simulink model "SimulinkAnalysisofCheetahTail"  (R2022a)
settings: Solver=ode4  StartTime=0.0  StopTime=1.5  FixedStep=0.001  RelTol=1e-3
undefined symbols (not defined in the file): B_cg_H, B_con_H, B_con_L, bar_len, cd_table, Cf, cl_table, g, gear_ratio, int_point_bar, int_point_tail, ITail, M_add, M_cg_H, M_cg_L, M_cg_W, Mb, Mm, Mt, psi3, rho, T_cg_H, T_fur_gap, T_length, T_width_major, T_width_minor, th2_initial, torque_constant, uncertainty_Forces, uncertainty_Position, Vf, windspeed
(part 14 of 21)

== matlab function SimulinkAnalysisofCheetahTail/Model/Forces/NonConstraintForceMatrix_tail_3 ==
  data: B_con_H parameter; B_con_L parameter; Cd input; Cl input; Q_tail_3 output; M_cg_H parameter; M_cg_L parameter; M_cg_W parameter; T_fur_gap parameter; T_length parameter; T_width_major parameter; T_width_minor parameter; area_tail_3_drag input; bar_len parameter; int_point_tail input; psi3 parameter; rho parameter; windspeed parameter; q input; dq input; ddq input
function Q_tail_3 = NonConstraintForceMatrix_tail_3(B_con_H,B_con_L,Cd,Cl,M_cg_H,M_cg_L,M_cg_W,T_fur_gap,T_length,T_width_major,T_width_minor,area_tail_3_drag,bar_len,int_point_tail,psi3,rho,windspeed,q,dq,ddq)
%#codegen
[x,y,z,phi1,th1,psi1,phi2,th2] = deal(q(1),q(2),q(3),q(4),q(5),q(6),q(7),q(8));
[dx,dy,dz,dphi1,dth1,dpsi1,dphi2,dth2] = deal(dq(1),dq(2),dq(3),dq(4),dq(5),dq(6),dq(7),dq(8));
[ddx,ddy,ddz,ddphi1,ddth1,ddpsi1,ddphi2,ddth2] = deal(ddq(1),ddq(2),ddq(3),ddq(4),ddq(5),ddq(6),ddq(7),ddq(8));
%    This function was generated by the Symbolic Math Toolbox version 9.0.
%    17-Feb-2022 11:27:23

t2 = cos(phi1);
t3 = cos(phi2);
t4 = cos(psi1);
t5 = cos(psi3);
t6 = cos(th1);
t7 = cos(th2);
t8 = sin(phi1);
t9 = sin(phi2);
t10 = sin(psi1);
t11 = sin(psi3);
t12 = sin(th1);
t13 = sin(th2);
t14 = M_cg_L+x;
t15 = M_cg_W+y;
t16 = M_cg_H+z;
t19 = -int_point_tail;
t27 = T_length./2.0;
t28 = bar_len./2.0;
t29 = int_point_tail./2.0;
t17 = B_con_L.*t6;
t18 = B_con_L.*t12;
t20 = t2.*t4;
t21 = t6.*t7;
t22 = t2.*t10;
t23 = t4.*t8;
t24 = t7.*t12;
t25 = t8.*t10;
t26 = t12.*t13;
t30 = B_con_H.*t2.*t6;
t32 = t6.*t14;
t33 = B_con_H.*t2.*t12;
t34 = B_con_H.*t6.*t8;
t37 = t12.*t14;
t39 = -t29;
t42 = t6.*t9.*t13;
t44 = t6.*t10.*t13;
t46 = t8.*t9.*t12;
t49 = t2.*t3.*t6;
t50 = T_length+bar_len+t19;
t53 = t2.*t6.*t9;
t54 = t3.*t6.*t8;
t56 = t2.*t6.*t13;
t57 = t3.*t6.*t13;
t59 = t4.*t6.*t13;
t62 = t3.*t8.*t12;
t63 = t6.*t8.*t9;
t68 = t2.*t6.*t15;
t70 = t2.*t6.*t16;
t73 = t6.*t8.*t15;
t74 = t2.*t12.*t16;
t75 = t6.*t8.*t16;
t77 = t8.*t12.*t15;
t105 = t5.*t6.*t8.*t13;
t111 = t6.*t8.*t11.*t13;
t31 = t4.*t17;
t35 = t4.*t18;
t36 = t10.*t17;
t38 = t10.*t18;
t40 = t2.*t26;
t41 = t3.*t26;
t43 = t9.*t24;
t45 = t10.*t24;
t47 = t12.*t25;
t48 = t9.*t26;
t51 = t2.*t21;
t52 = t4.*t21;
t55 = t12.*t20;
t58 = t3.*t24;
t60 = t4.*t24;
t61 = t10.*t21;
t64 = t12.*t22;
t65 = t12.*t23;
t66 = B_con_H.*t6.*t20;
t67 = t4.*t32;
t69 = B_con_H.*t6.*t22;
t71 = t4.*t37;
t72 = t10.*t32;
t76 = t10.*t37;
t78 = -t33;
t79 = -t34;
t81 = -t46;
t86 = t3.*t6.*t23;
t87 = t13.*t49;
t90 = t3.*t8.*t21;
t91 = t6.*t13.*t20;
t92 = t4.*t57;
t95 = t3.*t6.*t25;
t96 = t6.*t9.*t23;
t97 = t2.*t42;
t99 = t8.*t9.*t21;
t100 = t6.*t13.*t22;
t102 = t3.*t44;
t103 = t4.*t42;
t106 = t6.*t9.*t25;
t110 = t10.*t42;
t113 = -t59;
t116 = t6.*t16.*t20;
t117 = t6.*t15.*t23;
t118 = t6.*t16.*t22;
t119 = t6.*t15.*t25;
t120 = -t68;
t121 = -t73;
t122 = -t74;
t123 = -t75;
t124 = t3.*t20.*t21;
t125 = t3.*t21.*t22;
t126 = t9.*t20.*t21;
t127 = t9.*t21.*t22;
t133 = -t105;
t138 = t24+t56;
t165 = t27+t28+t39;
t80 = -t40;
t82 = -t47;
t83 = -t48;
t84 = t3.*t51;
t85 = t3.*t52;
t88 = t2.*t58;
t89 = t9.*t51;
t93 = t3.*t61;
t94 = t9.*t52;
t98 = t2.*t43;
t101 = t4.*t41;
t104 = t9.*t61;
t107 = -t51;
t108 = t10.*t41;
t109 = t4.*t48;
t112 = -t55;
t114 = -t61;
t115 = t10.*t48;
t129 = -t92;
t131 = -t99;
t136 = -t117;
t137 = -t119;
t139 = t22+t65;
t140 = t23+t64;
t141 = -t124;
t142 = -t125;
t149 = t5.*t138;
t153 = t11.*t138;
t157 = t53+t90;
t161 = t58+t87;
t162 = t60+t91;
t163 = t43+t97;
t164 = t45+t100;
t128 = -t84;
t130 = -t93;
t132 = -t104;
t134 = t4.*t83;
t135 = t10.*t83;
t143 = B_con_H.*t139;
t144 = B_con_H.*t140;
t145 = t21+t80;
t146 = t26+t107;
t147 = t20+t82;
t148 = t25+t112;
t150 = t3.*t139;
t151 = t3.*t140;
t152 = t7.*t140;
t154 = t9.*t139;
t155 = t9.*t140;
t156 = t13.*t140;
t166 = t15.*t139;
t167 = t15.*t140;
t168 = t16.*t139;
t169 = t16.*t140;
t175 = t5.*t13.*t139;
t177 = t11.*t13.*t139;
t185 = -t153;
t189 = t49+t131;
t190 = T_fur_gap.*t157;
t191 = T_fur_gap.*t161;
t192 = int_point_tail.*t157;
t193 = int_point_tail.*t161;
t200 = t5.*t162;
t201 = t11.*t162;
t202 = t5.*t163;
t203 = t5.*t164;
t204 = t11.*t163;
t205 = t11.*t164;
t228 = t42+t62+t98;
t231 = t57+t81+t88;
t232 = t54+t83+t89;
t266 = t96+t101+t141;
t268 = t106+t108+t142;
t282 = t157.*t165;
t283 = t161.*t165;
t158 = B_con_H.*t147;
t159 = B_con_H.*t148;
t160 = -t144;
t170 = t7.*t150;
t171 = t7.*t151;
t172 = t13.*t151;
t173 = t7.*t154;
t174 = t9.*t152;
t176 = t13.*t155;
t178 = t5.*t145;
t179 = t5.*t146;
t180 = t3.*t147;
t181 = t3.*t148;
t182 = t7.*t148;
t183 = t11.*t145;
t184 = t11.*t146;
t186 = t9.*t147;
t187 = t9.*t148;
t188 = t13.*t148;
t194 = t15.*t147;
t195 = t15.*t148;
t196 = -t167;
t197 = t16.*t147;
t198 = t16.*t148;
t199 = -t169;
t212 = t5.*t13.*t147;
t214 = t11.*t13.*t147;
t215 = -t177;
t221 = t5.*t189;
t222 = t11.*t189;
t223 = -t205;
t227 = t44+t152;
t229 = t114+t156;
t230 = t41+t63+t128;
t236 = t5.*t228;
t237 = t11.*t228;
t239 = T_fur_gap.*t231;
t240 = T_fur_gap.*t232;
t242 = int_point_tail.*t231;
t243 = int_point_tail.*t232;
t246 = -t5.*(t61-t156);
t249 = -t11.*(t61-t156);
t250 = t5.*t232;
t252 = t11.*t232;
t267 = t86+t126+t134;
t269 = t95+t127+t135;
t276 = T_fur_gap.*t266;
t277 = int_point_tail.*t266;
t278 = T_fur_gap.*t268;
t279 = int_point_tail.*t268;
t303 = t165.*t231;
t304 = t165.*t232;
t325 = t165.*t266;
t326 = t165.*t268;
t370 = t191+t193+t283;
t397 = t79+t120+t123+t190+t192+t282;
t206 = t7.*t180;
t207 = t7.*t181;
t208 = -t170;
t209 = t13.*t181;
t210 = t7.*t186;
t211 = t9.*t182;
t213 = t13.*t187;
t216 = -t178;
t217 = -t180;
t218 = -t184;
t219 = -t194;
t220 = -t195;
t226 = -t214;
t233 = t52+t188;
t234 = t5.*t227;
t235 = t11.*t227;
t238 = T_fur_gap.*t230;
t241 = int_point_tail.*t230;
t244 = t113+t182;
t251 = t12.*t230;
t254 = t130+t172;
t256 = t132+t176;
t257 = t2.*t6.*t230;
t258 = -t5.*(t59-t182);
t259 = t6.*t8.*t230;
t260 = -t11.*(t59-t182);
t262 = -T_fur_gap.*(t93-t172);
t264 = -int_point_tail.*(t93-t172);
t265 = t111+t221;
t270 = -t5.*(t104-t176);
t272 = -t11.*(t104-t176);
t274 = t5.*(t59-t182);
t280 = t133+t222;
t281 = t5.*t269;
t284 = t11.*t269;
t285 = t5.*t267;
t286 = t11.*t267;
t288 = t173+t181;
t290 = t179+t204;
t298 = -T_fur_gap.*(t170-t187);
t300 = -int_point_tail.*(t170-t187);
t302 = t165.*t230;
t305 = t149+t252;
t306 = t102+t171+t186;
t307 = t183+t236;
t311 = t185+t250;
t316 = -t165.*(t93-t172);
t333 = -t12.*(t153-t250);
t339 = -t2.*t6.*(t153-t250);
t340 = -t6.*t8.*(t153-t250);
t346 = t2.*t6.*(t153-t250);
t350 = -t165.*(t170-t187);
t395 = t240+t243+t304;
t396 = t230.*t370;
t401 = -t370.*(t153-t250);
t402 = t370.*(t153-t250);
t404 = -t230.*(t34+t68+t75-t190-t192-t282);
t408 = t17+t32+t77+t78+t122+t239+t242+t303;
t416 = (t153-t250).*(t34+t68+t75-t190-t192-t282);
t432 = t38+t69+t76+t118+t137+t278+t279+t326;
t433 = t35+t66+t71+t116+t136+t276+t277+t325;
t224 = -t206;
t225 = -t211;
t245 = t5.*t233;
t247 = t11.*t233;
t248 = -t234;
t253 = t85+t209;
t255 = t94+t213;
t273 = -t257;
t287 = t151+t210;
t289 = -t285;
t292 = t187+t208;
t294 = t5.*t288;
t296 = t11.*t288;
t301 = t202+t218;
t308 = T_fur_gap.*t306;
t309 = int_point_tail.*t306;
t310 = t129+t154+t207;
t313 = t216+t237;
t314 = t110+t174+t217;
t317 = t12.*t305;
t319 = t5.*t306.*windspeed;
t327 = t2.*t6.*t305;
t328 = t6.*t8.*t305;
t329 = t6.*t10.*t306;
t347 = t200+t286;
t348 = t203+t284;
t352 = t223+t281;
t354 = t140.*t306;
t355 = t235+t270;
t359 = t147.*t306;
t363 = t165.*t306;
t399 = t262+t264+t316;
t400 = t305.*t370;
t403 = t230.*t395;
t406 = t18+t30+t37+t70+t121+t238+t241+t302;
t413 = t305.*t395;
t414 = -t305.*(t34+t68+t75-t190-t192-t282);
t415 = -t395.*(t153-t250);
t417 = t395.*(t153-t250);
t420 = -t416;
t427 = -t306.*(T_fur_gap.*(t93-t172)+int_point_tail.*(t93-t172)+t165.*(t93-t172));
t431 = t306.*(T_fur_gap.*(t93-t172)+int_point_tail.*(t93-t172)+t165.*(t93-t172));
t439 = t230.*t408;
t452 = t305.*t408;
t453 = -t408.*(t153-t250);
t455 = t408.*(t153-t250);
t456 = t143+t168+t220+t298+t300+t350;
t462 = t306.*t432;
t261 = T_fur_gap.*t253;
t263 = int_point_tail.*t253;
t271 = t11.*t255;
t275 = t5.*t255;
t291 = t155+t224;
t293 = t5.*t287;
t295 = t11.*t287;
t312 = t103+t150+t225;
t315 = t165.*t253;
t318 = T_fur_gap.*t310;
t321 = int_point_tail.*t310;
t322 = T_fur_gap.*t314;
t324 = int_point_tail.*t314;
t331 = t5.*t314;
t334 = t11.*t314;
t336 = t11.*t310.*windspeed;
t337 = t19.*t310;
t338 = t4.*t6.*t310;
t341 = -t328;
t351 = t201+t289;
t353 = t175+t296;
t356 = t215+t294;
t358 = t139.*t310;
t360 = t248+t272;
t362 = t148.*t310;
t365 = t165.*t310;
t367 = t165.*t314;
t405 = -t403;
t418 = t157.*t406;
t419 = t161.*t406;
t428 = t231.*t406;
t429 = t232.*t406;
t434 = t5.*t230.*t406;
t435 = t11.*t230.*t406;
t441 = -t439;
t444 = t265.*t406;
t445 = -t406.*(t105-t222);
t447 = t290.*t406;
t448 = -t406.*(t184-t202);
t450 = t307.*t406;
t451 = -t406.*(t178-t237);
t454 = -t452;
t463 = t310.*t433;
t476 = t36+t72+t160+t199+t219+t308+t309+t363;
t478 = -t310.*(-t143-t168+t195+T_fur_gap.*(t170-t187)+int_point_tail.*(t170-t187)+t165.*(t170-t187));
t480 = t310.*(-t143-t168+t195+T_fur_gap.*(t170-t187)+int_point_tail.*(t170-t187)+t165.*(t170-t187));
t297 = T_fur_gap.*t291;
t299 = int_point_tail.*t291;
t320 = T_fur_gap.*t312;
t323 = int_point_tail.*t312;
t330 = t5.*t312;
t332 = t11.*t312;
t335 = -t318;
t342 = -t331;
t344 = -t336;
t345 = -t338;
t349 = t165.*t291;
t357 = t212+t295;
t361 = t226+t293;
t364 = t260+t275;
t366 = t165.*t312;
t368 = t271+t274;
t369 = -t365;
t372 = t246+t334;
t375 = t5.*windspeed.*(t334-t5.*(t61-t156));
t378 = t6.*t10.*(t334-t5.*(t61-t156));
t379 = -t5.*windspeed.*(t331+t11.*(t61-t156));
t384 = -t6.*t10.*(t331+t11.*(t61-t156));
t388 = t140.*(t334-t5.*(t61-t156));
t391 = t147.*(t334-t5.*(t61-t156));
t392 = -t140.*(t331+t11.*(t61-t156));
t394 = -t147.*(t331+t11.*(t61-t156));
t398 = t261+t263+t315;
t421 = t259+t358+t359;
t424 = t273+t354+t362;
t436 = -t428;
t437 = -t429;
t440 = -t435;
t443 = t322+t324+t367;
t446 = -t444;
t449 = -t447;
t459 = -(t334-t5.*(t61-t156)).*(T_fur_gap.*(t93-t172)+int_point_tail.*(t93-t172)+t165.*(t93-t172));
t461 = (t331+t11.*(t61-t156)).*(T_fur_gap.*(t93-t172)+int_point_tail.*(t93-t172)+t165.*(t93-t172));
t465 = -t463;
t482 = t432.*(t334-t5.*(t61-t156));
t485 = -t432.*(t331+t11.*(t61-t156));
t506 = -t476.*(t93-t172);
t507 = t476.*(t93-t172);
t508 = t268.*t476;
t510 = t291.*t476;
t518 = t5.*t306.*t476;
t519 = t11.*t306.*t476;
t520 = t314.*t476;
t522 = t348.*t476;
t524 = -t476.*(t205-t281);
t528 = t355.*t476;
t530 = -t476.*(t234+t11.*(t104-t176));
t532 = -t476.*(t214-t293);
t343 = -t332;
t371 = t247+t330;
t374 = t249+t342;
t385 = -t378;
t407 = t251+t329+t345;
t422 = ddy.*t421;
t423 = dy.*t421;
t425 = ddz.*t424;
t426 = dz.*t424;
t430 = t310.*t398;
t442 = t320+t323+t366;
t458 = t158+t196+t197+t297+t299+t349;
t464 = t306.*t443;
t477 = t31+t67+t159+t166+t198+t335+t337+t369;
t486 = -t482;
t493 = t443.*(t334-t5.*(t61-t156));
t500 = -t443.*(t331+t11.*(t61-t156));
t512 = -t510;
t521 = -t519;
t529 = t357.*t476;
t531 = -t528;
t373 = t245+t343;
t376 = t11.*t371.*windspeed;
t377 = t4.*t6.*t371;
t387 = t139.*t371;
t389 = t148.*t371;
t409 = ddx.*t407;
t410 = dx.*t407;
t438 = -t430;
t457 = t371.*t398;
t466 = t310.*t442;
t479 = t306.*t458;
t483 = t371.*t433;
t494 = t371.*t442;
t509 = t253.*t477;
t511 = t266.*t477;
t513 = -t371.*(-t143-t168+t195+T_fur_gap.*(t170-t187)+int_point_tail.*(t170-t187)+t165.*(t170-t187));
t515 = t458.*(t334-t5.*(t61-t156));
t516 = -t458.*(t331+t11.*(t61-t156));
t517 = -t477.*(t170-t187);
t523 = t312.*t477;
t525 = t5.*t310.*t477;
t526 = t11.*t310.*t477;
t533 = -t529;
t534 = t347.*t477;
t535 = t351.*t477;
t536 = t353.*t477;
t538 = -t477.*(t177-t294);
t539 = t477.*(t177-t294);
t540 = t364.*t477;
t541 = t368.*t477;
Q_tail_3 = ft_1({Cd,Cl,T_fur_gap,T_width_major,T_width_minor,area_tail_3_drag,ddphi1,ddphi2,ddth1,ddth2,ddx,ddy,ddz,dphi1,dphi2,dth1,dth2,dx,dy,dz,int_point_tail,rho,t10,t104,t105,t11,t12,t138,t139,t140,t143,t147,t148,t153,t156,t165,t168,t170,t172,t176,t178,t187,t190,t192,t195,t2,t205,t214,t222,t230,t232,t233,t234,t237,t250,t281,t282,t293,t305,t306,t310,t312,t314,t317,t319,t327,t331,t333,t334,t34,t340,t341,t344,t346,t370,t371,t373,t375,t376,t377,t379,t384,t385,t387,t388,t389,t391,t392,t394,t395,t396,t398,t4,t400,t402,t403,t404,t405,t406,t408,t409,t410,t413,t414,t415,t416,t417,t418,t419,t420,t422,t423,t425,t426,t428,t429,t431,t432,t433,t434,t436,t437,t438,t439,t440,t441,t442,t443,t444,t445,t446,t447,t448,t449,t450,t451,t452,t453,t454,t455,t457,t458,t459,t461,t462,t463,t464,t465,t466,t476,t477,t478,t479,t480,t482,t483,t485,t486,t493,t494,t5,t50,t500,t507,t508,t509,t510,t511,t512,t513,t515,t516,t517,t518,t520,t521,t522,t523,t524,t525,t526,t529,t530,t531,t532,t533,t534,t535,t536,t538,t539,t540,t541,t6,t61,t68,t75,t8,t93,th2,windspeed});
end
function Q_tail_3 = ft_1(ct)
Cd = ct{1};
Cl = ct{2};
T_fur_gap = ct{3};
T_width_major = ct{4};
T_width_minor = ct{5};
area_tail_3_drag = ct{6};
ddphi1 = ct{7};
ddphi2 = ct{8};
ddth1 = ct{9};
ddth2 = ct{10};
ddx = ct{11};
ddy = ct{12};
ddz = ct{13};
dphi1 = ct{14};
dphi2 = ct{15};
dth1 = ct{16};
dth2 = ct{17};
dx = ct{18};
dy = ct{19};
dz = ct{20};
int_point_tail = ct{21};
rho = ct{22};
t10 = ct{23};
t104 = ct{24};
t105 = ct{25};
t11 = ct{26};
t12 = ct{27};
t138 = ct{28};
t139 = ct{29};
t140 = ct{30};
t143 = ct{31};
t147 = ct{32};
t148 = ct{33};
t153 = ct{34};
t156 = ct{35};
t165 = ct{36};
t168 = ct{37};
t170 = ct{38};
t172 = ct{39};
t176 = ct{40};
t178 = ct{41};
t187 = ct{42};
t190 = ct{43};
t192 = ct{44};
t195 = ct{45};
t2 = ct{46};
t205 = ct{47};
t214 = ct{48};
t222 = ct{49};
t230 = ct{50};
t232 = ct{51};
t233 = ct{52};
t234 = ct{53};
t237 = ct{54};
t250 = ct{55};
t281 = ct{56};
t282 = ct{57};
t293 = ct{58};
t305 = ct{59};
t306 = ct{60};
t310 = ct{61};
t312 = ct{62};
t314 = ct{63};
t317 = ct{64};
t319 = ct{65};
t327 = ct{66};
t331 = ct{67};
t333 = ct{68};
t334 = ct{69};
t34 = ct{70};
t340 = ct{71};
t341 = ct{72};
t344 = ct{73};
t346 = ct{74};
t370 = ct{75};
t371 = ct{76};
t373 = ct{77};
t375 = ct{78};
t376 = ct{79};
t377 = ct{80};
t379 = ct{81};
t384 = ct{82};
t385 = ct{83};
t387 = ct{84};
t388 = ct{85};
t389 = ct{86};
t391 = ct{87};
t392 = ct{88};
t394 = ct{89};
t395 = ct{90};
t396 = ct{91};
t398 = ct{92};
t4 = ct{93};
t400 = ct{94};
t402 = ct{95};
t403 = ct{96};
t404 = ct{97};
t405 = ct{98};
t406 = ct{99};
t408 = ct{100};
t409 = ct{101};
t410 = ct{102};
t413 = ct{103};
t414 = ct{104};
t415 = ct{105};
t416 = ct{106};
t417 = ct{107};
t418 = ct{108};
t419 = ct{109};
t420 = ct{110};
t422 = ct{111};
t423 = ct{112};
t425 = ct{113};
t426 = ct{114};
t428 = ct{115};
t429 = ct{116};
t431 = ct{117};
t432 = ct{118};
t433 = ct{119};
t434 = ct{120};
t436 = ct{121};
t437 = ct{122};
t438 = ct{123};
t439 = ct{124};
t440 = ct{125};
t441 = ct{126};
t442 = ct{127};
t443 = ct{128};
t444 = ct{129};
t445 = ct{130};
t446 = ct{131};
t447 = ct{132};
t448 = ct{133};
t449 = ct{134};
t450 = ct{135};
t451 = ct{136};
t452 = ct{137};
t453 = ct{138};
t454 = ct{139};
t455 = ct{140};
t457 = ct{141};
t458 = ct{142};
t459 = ct{143};
t461 = ct{144};
t462 = ct{145};
t463 = ct{146};
t464 = ct{147};
t465 = ct{148};
t466 = ct{149};
t476 = ct{150};
t477 = ct{151};
t478 = ct{152};
t479 = ct{153};
t480 = ct{154};
t482 = ct{155};
t483 = ct{156};
t485 = ct{157};
t486 = ct{158};
t493 = ct{159};
t494 = ct{160};
t5 = ct{161};
t50 = ct{162};
t500 = ct{163};
t507 = ct{164};
t508 = ct{165};
t509 = ct{166};
t510 = ct{167};
t511 = ct{168};
t512 = ct{169};
t513 = ct{170};
t515 = ct{171};
t516 = ct{172};
t517 = ct{173};
t518 = ct{174};
t520 = ct{175};
t521 = ct{176};
t522 = ct{177};
t523 = ct{178};
t524 = ct{179};
t525 = ct{180};
t526 = ct{181};
t529 = ct{182};
t530 = ct{183};
t531 = ct{184};
t532 = ct{185};
t533 = ct{186};
t534 = ct{187};
t535 = ct{188};
t536 = ct{189};
t538 = ct{190};
t539 = ct{191};
t540 = ct{192};
t541 = ct{193};
t6 = ct{194};
t61 = ct{195};
t68 = ct{196};
t75 = ct{197};
t8 = ct{198};
t93 = ct{199};
th2 = ct{200};
windspeed = ct{201};
t380 = t11.*t373.*windspeed;
t381 = -t376;
t382 = t4.*t6.*t373;
t383 = -t377;
t390 = t139.*t373;
t393 = t148.*t373;
t411 = -t409;
t412 = -t410;
t460 = t373.*t398;
t467 = -t466;
t472 = -ddx.*(t377+t12.*(t153-t250)+t6.*t10.*(t331+t11.*(t61-t156)));
t473 = -dx.*(t377+t12.*(t153-t250)+t6.*t10.*(t331+t11.*(t61-t156)));
t474 = ddx.*(t377+t12.*(t153-t250)+t6.*t10.*(t331+t11.*(t61-t156)));
t475 = dx.*(t377+t12.*(t153-t250)+t6.*t10.*(t331+t11.*(t61-t156)));
t481 = -t479;
t487 = t373.*t433;
t488 = -t483;
t489 = t340+t387+t394;
t495 = -ddy.*(-t387+t147.*(t331+t11.*(t61-t156))+t6.*t8.*(t153-t250));
t497 = -dy.*(-t387+t147.*(t331+t11.*(t61-t156))+t6.*t8.*(t153-t250));
t499 = t346+t389+t392;
t501 = t373.*t442;
t502 = -t494;
t514 = -t373.*(-t143-t168+t195+T_fur_gap.*(t170-t187)+int_point_tail.*(t170-t187)+t165.*(t170-t187));
t527 = -t525;
t537 = -t535;
t542 = -t541;
t543 = t396+t419+t431+t438+t507+t509;
t548 = t436+t441+t462+t465+t508+t511;
t549 = -ddth1.*(t428+t439-t462+t463-t508-t511);
t550 = -dth1.*(t428+t439-t462+t463-t508-t511);
t552 = t402+t448+t457+t461+t531+t540;
t554 = -ddphi2.*(t403+t429-t464+t466-t520-t523);
t555 = -dphi2.*(t403+t429-t464+t466-t520-t523);
t561 = -ddphi1.*(-t418+t478+t479+t510+t230.*(t34+t68+t75-t190-t192-t282)+t477.*(t170-t187));
t562 = -dphi1.*(-t418+t478+t479+t510+t230.*(t34+t68+t75-t190-t192-t282)+t477.*(t170-t187));
t563 = ddphi1.*(-t418+t478+t479+t510+t230.*(t34+t68+t75-t190-t192-t282)+t477.*(t170-t187));
t564 = dphi1.*(-t418+t478+t479+t510+t230.*(t34+t68+t75-t190-t192-t282)+t477.*(t170-t187));
t569 = -ddphi2.*(t415-t434+t494-t518+t525+t443.*(t331+t11.*(t61-t156)));
t570 = -dphi2.*(t415-t434+t494-t518+t525+t443.*(t331+t11.*(t61-t156)));
t577 = -ddth1.*(-t450+t453+t483+t535+t432.*(t331+t11.*(t61-t156))+t476.*(t205-t281));
t578 = -dth1.*(-t450+t453+t483+t535+t432.*(t331+t11.*(t61-t156))+t476.*(t205-t281));
t580 = -ddphi1.*(-t515+t529-t536+t305.*(t34+t68+t75-t190-t192-t282)+t406.*(t105-t222)+t373.*(-t143-t168+t195+T_fur_gap.*(t170-t187)+int_point_tail.*(t170-t187)+t165.*(t170-t187)));
t581 = -dphi1.*(-t515+t529-t536+t305.*(t34+t68+t75-t190-t192-t282)+t406.*(t105-t222)+t373.*(-t143-t168+t195+T_fur_gap.*(t170-t187)+int_point_tail.*(t170-t187)+t165.*(t170-t187)));
t582 = t420+t446+t513+t516+t532+t539;
t583 = -ddphi1.*(t416+t444+t538+t458.*(t331+t11.*(t61-t156))+t476.*(t214-t293)+t371.*(-t143-t168+t195+T_fur_gap.*(t170-t187)+int_point_tail.*(t170-t187)+t165.*(t170-t187)));
t584 = -dphi1.*(t416+t444+t538+t458.*(t331+t11.*(t61-t156))+t476.*(t214-t293)+t371.*(-t143-t168+t195+T_fur_gap.*(t170-t187)+int_point_tail.*(t170-t187)+t165.*(t170-t187)));
t386 = -t380;
t468 = t317+t382+t385;
t471 = t333+t383+t384;
t484 = t327+t388+t393;
t490 = t341+t390+t391;
t503 = ddz.*t499;
t504 = dz.*t499;
t505 = -t501;
t544 = ddth2.*t543;
t545 = dth2.*t543;
t551 = t405+t437+t464+t467+t520+t523;
t553 = t400+t449+t459+t460+t530+t542;
t556 = ddth2.*t552;
t557 = -ddth2.*(-t400+t447-t460+t541+t476.*(t234+t11.*(t104-t176))+(t334-t5.*(t61-t156)).*(T_fur_gap.*(t93-t172)+int_point_tail.*(t93-t172)+t165.*(t93-t172)));
t558 = dth2.*t552;
t559 = -dth2.*(-t400+t447-t460+t541+t476.*(t234+t11.*(t104-t176))+(t334-t5.*(t61-t156)).*(T_fur_gap.*(t93-t172)+int_point_tail.*(t93-t172)+t165.*(t93-t172)));
t560 = t404+t418+t480+t481+t512+t517;
t568 = t417+t434+t500+t502+t518+t527;
t571 = t451+t454+t486+t487+t522+t534;
t572 = -ddth1.*(t452+t482-t487-t522-t534+t406.*(t178-t237));
t573 = -dth1.*(t452+t482-t487-t522-t534+t406.*(t178-t237));
t574 = ddth1.*(t452+t482-t487-t522-t534+t406.*(t178-t237));
t575 = dth1.*(t452+t482-t487-t522-t534+t406.*(t178-t237));
t576 = t450+t455+t485+t488+t524+t537;
t579 = t414+t445+t514+t515+t533+t536;
t469 = ddx.*t468;
t470 = dx.*t468;
t491 = ddz.*t484;
t492 = dz.*t484;
t496 = ddy.*t490;
t498 = dy.*t490;
t546 = -t544;
t547 = -t545;
t565 = t413+t440+t493+t505+t521+t526;
t594 = t474+t495+t503+t556+t569+t577+t583;
t600 = t379+t381+t475+t497+t504+t558+t570+t578+t584;
t602 = -1.0./(t376+t473-t504-t558+dy.*(-t387+t147.*(t331+t11.*(t61-t156))+t6.*t8.*(t153-t250))+dphi2.*(t415-t434+t494-t518+t525+t443.*(t331+t11.*(t61-t156)))+dphi1.*(t416+t444+t538+t458.*(t331+t11.*(t61-t156))+t476.*(t214-t293)+t371.*(-t143-t168+t195+T_fur_gap.*(t170-t187)+int_point_tail.*(t170-t187)+t165.*(t170-t187)))+dth1.*(-t450+t453+t483+t535+t432.*(t331+t11.*(t61-t156))+t476.*(t205-t281))+t5.*windspeed.*(t331+t11.*(t61-t156)));
t566 = ddphi2.*t565;
t567 = dphi2.*t565;
t585 = t411+t422+t425+t546+t549+t554+t563;
t588 = t319+t344+t412+t423+t426+t547+t550+t555+t564;
t595 = abs(t594);
t601 = abs(t600);
t586 = abs(t585);
t589 = abs(t588);
t591 = t469+t491+t496+t557+t566+t574+t580;
t596 = t595.^2;
t597 = t375+t386+t470+t492+t498+t559+t567+t575+t581;
t603 = t601.^2;
t604 = t588.*t602;
t587 = t586.^2;
t590 = t589.^2;
t592 = abs(t591);
t598 = abs(t597);
t605 = atan(t604);
t593 = t592.^2;
t599 = t598.^2;
t606 = -t605;
t607 = t606+th2;
t609 = t587+t593+t596;
t612 = t590+t599+t603;
t608 = cos(t607);
t610 = sqrt(t609);
t613 = sqrt(t612);
t611 = (T_width_major.*T_width_minor.*rho.*t50.*t610.*pi)./2.0e+1;
t614 = 1.0./t613;
t615 = (Cd.*area_tail_3_drag.*rho.*t608.*t612)./2.0;
t616 = (Cl.*T_width_major.*T_width_minor.*rho.*t588.*t608.*t613.*pi)./2.0;
t617 = Cl.*T_width_major.*T_width_minor.*rho.*t588.*t608.*t613.*pi.*3.061616997868383e-17;
t618 = (Cl.*T_width_major.*T_width_minor.*rho.*t138.*t597.*t608.*t613.*pi)./2.0;
t619 = Cl.*T_width_major.*T_width_minor.*rho.*t608.*t613.*pi.*(t376+t473-t504-t558+dy.*(-t387+t147.*(t331+t11.*(t61-t156))+t6.*t8.*(t153-t250))+dphi2.*(t415-t434+t494-t518+t525+t443.*(t331+t11.*(t61-t156)))+dphi1.*(t416+t444+t538+t458.*(t331+t11.*(t61-t156))+t476.*(t214-t293)+t371.*(-t143-t168+t195+T_fur_gap.*(t170-t187)+int_point_tail.*(t170-t187)+t165.*(t170-t187)))+dth1.*(-t450+t453+t483+t535+t432.*(t331+t11.*(t61-t156))+t476.*(t205-t281))+t5.*windspeed.*(t331+t11.*(t61-t156))).*(-1.0./2.0);
t620 = (Cl.*T_width_major.*T_width_minor.*rho.*t233.*t597.*t608.*t613.*pi)./2.0;
t621 = Cl.*T_width_major.*T_width_minor.*rho.*t597.*t608.*t613.*pi.*(t61-t156).*(-1.0./2.0);
et1 = Cl.*T_width_major.*T_width_minor.*rho.*t608.*t613.*pi.*(t376+t473-t504-t558+dy.*(-t387+t147.*(t331+t11.*(t61-t156))+t6.*t8.*(t153-t250))+dphi2.*(t415-t434+t494-t518+t525+t443.*(t331+t11.*(t61-t156)))+dphi1.*(t416+t444+t538+t458.*(t331+t11.*(t61-t156))+t476.*(t214-t293)+t371.*(-t143-t168+t195+T_fur_gap.*(t170-t187)+int_point_tail.*(t170-t187)+t165.*(t170-t187)))+dth1.*(-t450+t453+t483+t535+t432.*(t331+t11.*(t61-t156))+t476.*(t205-t281))+t5.*windspeed.*(t331+t11.*(t61-t156)));
et2 = -3.061616997868383e-17;
t622 = et1.*et2;
et3 = Cl.*T_width_major.*T_width_minor.*rho.*t608.*t613.*pi.*(t376+t473-t504-t558+dy.*(-t387+t147.*(t331+t11.*(t61-t156))+t6.*t8.*(t153-t250))+dphi2.*(t415-t434+t494-t518+t525+t443.*(t331+t11.*(t61-t156)))+dphi1.*(t416+t444+t538+t458.*(t331+t11.*(t61-t156))+t476.*(t214-t293)+t371.*(-t143-t168+t195+T_fur_gap.*(t170-t187)+int_point_tail.*(t170-t187)+t165.*(t170-t187)))+dth1.*(-t450+t453+t483+t535+t432.*(t331+t11.*(t61-t156))+t476.*(t205-t281))+t5.*windspeed.*(t331+t11.*(t61-t156)));
et4 = 3.061616997868383e-17;
t623 = et3.*et4;
t624 = t611+t615;
t628 = t617+t619;
t629 = t616+t623;
t625 = t230.*t588.*t614.*t624;
t626 = t306.*t588.*t614.*t624;
t627 = t310.*t588.*t614.*t624;
t630 = t230.*t628;
t631 = t232.*t629;
t633 = t306.*t628;
t634 = t310.*t628;
t635 = t312.*t629;
t636 = t314.*t629;
t638 = t138.*t597.*t614.*t624;
t640 = t233.*t597.*t614.*t624;
t641 = -t597.*t614.*t624.*(t61-t156);
t642 = -t232.*t614.*t624.*(t376+t473-t504-t558+dy.*(-t387+t147.*(t331+t11.*(t61-t156))+t6.*t8.*(t153-t250))+dphi2.*(t415-t434+t494-t518+t525+t443.*(t331+t11.*(t61-t156)))+dphi1.*(t416+t444+t538+t458.*(t331+t11.*(t61-t156))+t476.*(t214-t293)+t371.*(-t143-t168+t195+T_fur_gap.*(t170-t187)+int_point_tail.*(t170-t187)+t165.*(t170-t187)))+dth1.*(-t450+t453+t483+t535+t432.*(t331+t11.*(t61-t156))+t476.*(t205-t281))+t5.*windspeed.*(t331+t11.*(t61-t156)));
t643 = -t312.*t614.*t624.*(t376+t473-t504-t558+dy.*(-t387+t147.*(t331+t11.*(t61-t156))+t6.*t8.*(t153-t250))+dphi2.*(t415-t434+t494-t518+t525+t443.*(t331+t11.*(t61-t156)))+dphi1.*(t416+t444+t538+t458.*(t331+t11.*(t61-t156))+t476.*(t214-t293)+t371.*(-t143-t168+t195+T_fur_gap.*(t170-t187)+int_point_tail.*(t170-t187)+t165.*(t170-t187)))+dth1.*(-t450+t453+t483+t535+t432.*(t331+t11.*(t61-t156))+t476.*(t205-t281))+t5.*windspeed.*(t331+t11.*(t61-t156)));
t644 = -t314.*t614.*t624.*(t376+t473-t504-t558+dy.*(-t387+t147.*(t331+t11.*(t61-t156))+t6.*t8.*(t153-t250))+dphi2.*(t415-t434+t494-t518+t525+t443.*(t331+t11.*(t61-t156)))+dphi1.*(t416+t444+t538+t458.*(t331+t11.*(t61-t156))+t476.*(t214-t293)+t371.*(-t143-t168+t195+T_fur_gap.*(t170-t187)+int_point_tail.*(t170-t187)+t165.*(t170-t187)))+dth1.*(-t450+t453+t483+t535+t432.*(t331+t11.*(t61-t156))+t476.*(t205-t281))+t5.*windspeed.*(t331+t11.*(t61-t156)));
t645 = t314.*t614.*t624.*(t376+t473-t504-t558+dy.*(-t387+t147.*(t331+t11.*(t61-t156))+t6.*t8.*(t153-t250))+dphi2.*(t415-t434+t494-t518+t525+t443.*(t331+t11.*(t61-t156)))+dphi1.*(t416+t444+t538+t458.*(t331+t11.*(t61-t156))+t476.*(t214-t293)+t371.*(-t143-t168+t195+T_fur_gap.*(t170-t187)+int_point_tail.*(t170-t187)+t165.*(t170-t187)))+dth1.*(-t450+t453+t483+t535+t432.*(t331+t11.*(t61-t156))+t476.*(t205-t281))+t5.*windspeed.*(t331+t11.*(t61-t156)));
t632 = -t630;
t637 = -t635;
t639 = -t638;
t647 = t621+t633+t636;
t650 = t627+t640+t643;
t651 = t626+t641+t645;
t646 = t618+t631+t632;
t648 = t620+t634+t637;
t649 = t625+t639+t642;
et5 = -t12.*t646+t12.*(-t625+t638+t232.*t614.*t624.*(t376+t473-t504-t558+dy.*(-t387+t147.*(t331+t11.*(t61-t156))+t6.*t8.*(t153-t250))+dphi2.*(t415-t434+t494-t518+t525+t443.*(t331+t11.*(t61-t156)))+dphi1.*(t416+t444+t538+t458.*(t331+t11.*(t61-t156))+t476.*(t214-t293)+t371.*(-t143-t168+t195+T_fur_gap.*(t170-t187)+int_point_tail.*(t170-t187)+t165.*(t170-t187)))+dth1.*(-t450+t453+t483+t535+t432.*(t331+t11.*(t61-t156))+t476.*(t205-t281))+t5.*windspeed.*(t331+t11.*(t61-t156))))-t4.*t6.*t648+t4.*t6.*t650;
et6 = t6.*t10.*t647-t6.*t10.*t651;
et7 = -t139.*t648+t139.*t650-t147.*t647+t147.*t651;
et8 = -t6.*t8.*(-t625+t638+t232.*t614.*t624.*(t376+t473-t504-t558+dy.*(-t387+t147.*(t331+t11.*(t61-t156))+t6.*t8.*(t153-t250))+dphi2.*(t415-t434+t494-t518+t525+t443.*(t331+t11.*(t61-t156)))+dphi1.*(t416+t444+t538+t458.*(t331+t11.*(t61-t156))+t476.*(t214-t293)+t371.*(-t143-t168+t195+T_fur_gap.*(t170-t187)+int_point_tail.*(t170-t187)+t165.*(t170-t187)))+dth1.*(-t450+t453+t483+t535+t432.*(t331+t11.*(t61-t156))+t476.*(t205-t281))+t5.*windspeed.*(t331+t11.*(t61-t156))))+t6.*t8.*t646;
et9 = -t140.*t647+t140.*t651-t148.*t648+t148.*t650+t2.*t6.*(-t625+t638+t232.*t614.*t624.*(t376+t473-t504-t558+dy.*(-t387+t147.*(t331+t11.*(t61-t156))+t6.*t8.*(t153-t250))+dphi2.*(t415-t434+t494-t518+t525+t443.*(t331+t11.*(t61-t156)))+dphi1.*(t416+t444+t538+t458.*(t331+t11.*(t61-t156))+t476.*(t214-t293)+t371.*(-t143-t168+t195+T_fur_gap.*(t170-t187)+int_point_tail.*(t170-t187)+t165.*(t170-t187)))+dth1.*(-t450+t453+t483+t535+t432.*(t331+t11.*(t61-t156))+t476.*(t205-t281))+t5.*windspeed.*(t331+t11.*(t61-t156))));
et10 = -t2.*t6.*t646;
et11 = t646.*(t34+t68+t75-t190-t192-t282)-t458.*t647+t458.*t651;
et12 = -(-t625+t638+t232.*t614.*t624.*(t376+t473-t504-t558+dy.*(-t387+t147.*(t331+t11.*(t61-t156))+t6.*t8.*(t153-t250))+dphi2.*(t415-t434+t494-t518+t525+t443.*(t331+t11.*(t61-t156)))+dphi1.*(t416+t444+t538+t458.*(t331+t11.*(t61-t156))+t476.*(t214-t293)+t371.*(-t143-t168+t195+T_fur_gap.*(t170-t187)+int_point_tail.*(t170-t187)+t165.*(t170-t187)))+dth1.*(-t450+t453+t483+t535+t432.*(t331+t11.*(t61-t156))+t476.*(t205-t281))+t5.*windspeed.*(t331+t11.*(t61-t156)))).*(t34+t68+t75-t190-t192-t282);
et13 = t648.*(-t143-t168+t195+T_fur_gap.*(t170-t187)+int_point_tail.*(t170-t187)+t165.*(t170-t187))-t650.*(-t143-t168+t195+T_fur_gap.*(t170-t187)+int_point_tail.*(t170-t187)+t165.*(t170-t187));
et14 = -t408.*t646-t432.*t647+t433.*t648+t432.*t651-t433.*t650;
et15 = t408.*(-t625+t638+t232.*t614.*t624.*(t376+t473-t504-t558+dy.*(-t387+t147.*(t331+t11.*(t61-t156))+t6.*t8.*(t153-t250))+dphi2.*(t415-t434+t494-t518+t525+t443.*(t331+t11.*(t61-t156)))+dphi1.*(t416+t444+t538+t458.*(t331+t11.*(t61-t156))+t476.*(t214-t293)+t371.*(-t143-t168+t195+T_fur_gap.*(t170-t187)+int_point_tail.*(t170-t187)+t165.*(t170-t187)))+dth1.*(-t450+t453+t483+t535+t432.*(t331+t11.*(t61-t156))+t476.*(t205-t281))+t5.*windspeed.*(t331+t11.*(t61-t156))));
et16 = -t395.*t646+t442.*t648-t443.*t647-t442.*t650+t443.*t651;
et17 = t395.*(-t625+t638+t232.*t614.*t624.*(t376+t473-t504-t558+dy.*(-t387+t147.*(t331+t11.*(t61-t156))+t6.*t8.*(t153-t250))+dphi2.*(t415-t434+t494-t518+t525+t443.*(t331+t11.*(t61-t156)))+dphi1.*(t416+t444+t538+t458.*(t331+t11.*(t61-t156))+t476.*(t214-t293)+t371.*(-t143-t168+t195+T_fur_gap.*(t170-t187)+int_point_tail.*(t170-t187)+t165.*(t170-t187)))+dth1.*(-t450+t453+t483+t535+t432.*(t331+t11.*(t61-t156))+t476.*(t205-t281))+t5.*windspeed.*(t331+t11.*(t61-t156))));
et18 = -t370.*t646-t398.*t648+t398.*t650+t647.*(T_fur_gap.*(t93-t172)+int_point_tail.*(t93-t172)+t165.*(t93-t172))-t651.*(T_fur_gap.*(t93-t172)+int_point_tail.*(t93-t172)+t165.*(t93-t172));
et19 = t370.*(-t625+t638+t232.*t614.*t624.*(t376+t473-t504-t558+dy.*(-t387+t147.*(t331+t11.*(t61-t156))+t6.*t8.*(t153-t250))+dphi2.*(t415-t434+t494-t518+t525+t443.*(t331+t11.*(t61-t156)))+dphi1.*(t416+t444+t538+t458.*(t331+t11.*(t61-t156))+t476.*(t214-t293)+t371.*(-t143-t168+t195+T_fur_gap.*(t170-t187)+int_point_tail.*(t170-t187)+t165.*(t170-t187)))+dth1.*(-t450+t453+t483+t535+t432.*(t331+t11.*(t61-t156))+t476.*(t205-t281))+t5.*windspeed.*(t331+t11.*(t61-t156))));
Q_tail_3 = [et5+et6;et7+et8;et9+et10;et11+et12+et13;et14+et15;t476.*t648+t477.*t647-t476.*t650-t477.*t651;et16+et17;et18+et19];
end
